simulink subsystem "PieroAJ_Model"  (R2023b)
settings: Solver=VariableStepAuto  StartTime=0.0  StopTime=10.0  RelTol=1e-3
settings Model: Creator=USUARIO  LastModifiedBy=USUARIO

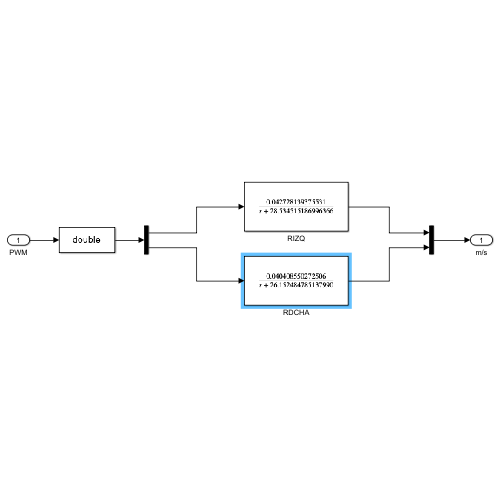
[thumbnail: Simulink's stored preview of the top-level diagram]
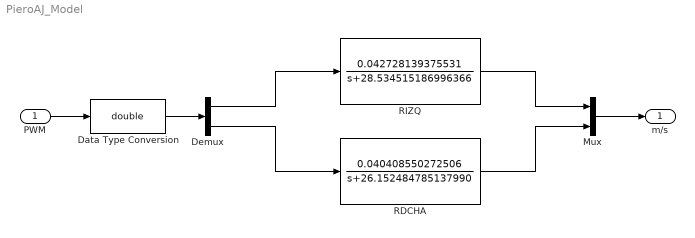
== system PieroAJ_Model ==
  PWM : Inport
  Data Type Conversion : DataTypeConversion  OutDataTypeStr=double  SaturateOnIntegerOverflow=off  RndMeth=Floor
  Demux : Demux  Outputs=2
  Mux : Mux  Inputs=2
  RDCHA : TransferFcn  Numerator=[0.040408550272506]  Denominator=[1 26.152484785137990]
  RIZQ : TransferFcn  Numerator=[0.042728139375531]  Denominator=[1 28.534515186996366]
  m/s : Outport
  wires:
  PWM/1 -> Data Type Conversion/1
  Data Type Conversion/1 -> Demux/1
  Mux/1 -> m/s/1
  Demux/1 -> RIZQ/1
  RIZQ/1 -> Mux/1
  RDCHA/1 -> Mux/2
  Demux/2 -> RDCHA/1
